simulink model "sim_sil_target_TrapezoidalCommutation_s32k1xx"  (Simulink 9.0)
settings: Solver=FixedStepDiscrete  StartTime=0.0  StopTime=12  FixedStep=1  RelTol=1e-3  EnableMultiTasking=on
InitFcn:
  | mbd_s32k_consistency_checks(bdroot(gcs));
undefined symbols (not defined in the file): LQFP
libraries: mbd_s32k1xx_ec_toolbox x1
settings Model: Creator=NXP MBDT Team  LastModifiedBy=nxf35172
settings DataIOCC: ExternalInput=off  InitialState=off  LimitDataPoints=on  SaveOutput=off  SignalLogging=off  SaveTime=off
settings OptimizationCC: DefaultParameterBehavior=Inlined  EnhancedBackFolding=on  PassReuseOutputArgsAs=Individual arguments  LifeSpan=auto  OptimizeBlockOrder=speed  DifferentSizesBufferReuse=on
settings DebuggingCC: UnderspecifiedInitializationDetection=Simplified  MergeDetectMultiDrivingBlocksExec=error  SolverPrmCheckMsg=warning  InheritedTsInSrcMsg=none  SingleTaskRateTransMsg=error  ParameterTunabilityLossMsg=error  UnconnectedInputMsg=error  UnconnectedOutputMsg=error  UnconnectedLineMsg=error  AllowSymbolicDim=off  UnknownTsInhSupMsg=error
settings HardwareCC: ProdIntDivRoundTo=Zero  ProdEndianess=LittleEndian  ProdHWDeviceType=Generic->Custom
settings SFSimCC: MATLABDynamicMemAlloc=off
settings RTWCC: SystemTargetFile=mbd_s32k.tlc  MakeCommand=mbd_s32k_make_rtw COPY_MDLREF_INCLUDES=0  TemplateMakefile=mbd_s32k.tmf  Description=Model Based Design Toolbox S32K1xx Code Generation Target  GenerateReport=on  IncludeHyperlinkInReport=on  LaunchReport=on  PortableWordSizes=on  GenerateTraceInfo=on  GenerateTraceReport=on  GenerateTraceReportSl=on  GenerateTraceReportSf=on  GenerateTraceReportEml=on
settings CodeAppCC: ForceParamTrailComments=on  IgnoreCustomStorageClasses=off  MaxIdLength=63  OperatorAnnotations=on  SimulinkDataObjDesc=on  SFDataObjDesc=on  InsertBlockDesc=on  StateflowObjectComments=off
settings STFCustomTargetCC: MultiwordLength=256  GenerateSampleERTMain=on  CombineOutputUpdateFcns=on  SuppressErrorStatus=on  ERTCustomFileBanners=on  SupportAbsoluteTime=off  SupportContinuousTime=off  SupportNonInlinedSFcns=off  RemoveResetFunc=on  MATLABClassNameForMDSCustomization=Simulink.SoftwareTarget.ERTCustomization  GRTInterface=off  SystemTargetFile=mbd_s32k.tlc
settings ERTTargetCC: GenerateSampleERTMain=on  ParMdlRefBuildCompliant=off  CompOptLevelCompliant=off  ConcurrentExecutionCompliant=off  SuppressErrorStatus=on  SupportAbsoluteTime=off  ModelStepFunctionPrototypeControlCompliant=off  CPPClassGenCompliant=off  UseToolchainInfoCompliant=off  InlinedParameterPlacement=NonHierarchical  ERTCustomFileTemplate=example_file_process.tlc

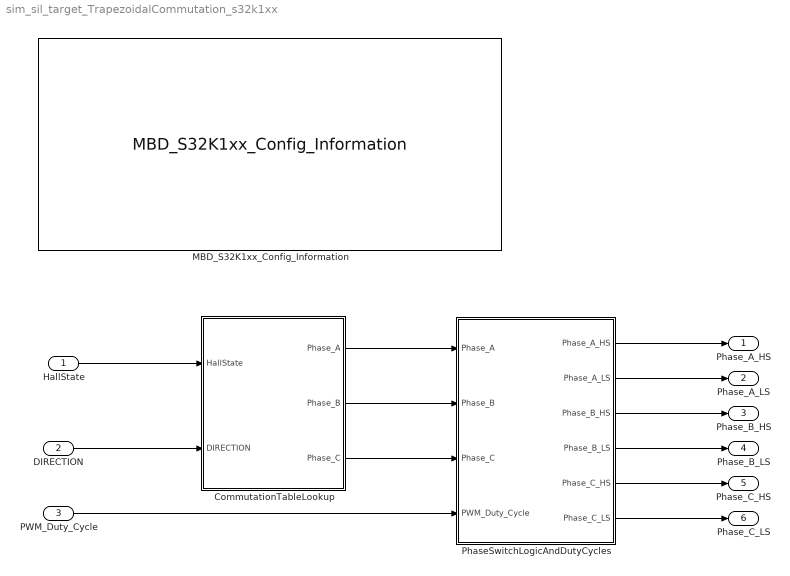
== system sim_sil_target_TrapezoidalCommutation_s32k1xx ==
  HallState : Inport
  DIRECTION : Inport  Port=2
  PWM_Duty_Cycle : Inport  Port=3
  CommutationTableLookup : Stateflow chart  TreatAsAtomicUnit=on
  MBD_S32K1xx_Config_Information : mbd_s32k1xx_ec_toolbox/MBD_S32K1xx_Config_Information  mbdt_ver=0  disp_str=|  config_params=target_mcu::S32K144-64KB_SRAM;;mcu_target_package::100-pin;;mcu_system_clock_freq::80;;mcu_xtal_freq::External 8;;mcu_steptick_timer::LPIT Channel 0;;mcu_steptick_prio::15;;ds_import_enable::on;;target_compiler::GCC;;target_memory::FLASH;;gcc_target_compile_opts::-c -mcpu=cortex-m4 -mthumb -mfloat-abi=hard -mfpu=fpv4-sp-d16 -O1 -g -gstrict-dwarf;;gcc_target_assemble_opts::-mcpu=cortex-m4 -mthumb -mfloat-abi=hard -mfpu=fpv4-sp-d16 -g;;gcc_target_link_opts::-mcpu=cortex-m4 -mthumb -mfloat-abi=hard -mfpu=fpv4-sp-d16;;gcc_target_lib_opts::;;gcc_target_default_lcf::on;;gcc_target_user_lcf::S32K144_64_flash.ld;;ghs_target_compile_opts::-cpu=cortexm4f -thumb -fpu=vfpv4_d16 -fsingle -Ogeneral -Wundef -Wimplicit-int -Wshadow -Wtrigraphs --no_commons --gnu_asm -gnu99 -gdwarf-2 -G ;;ghs_target_assemble_opts::-cpu=cortexm4f -fpu=vfpv4_d16;;ghs_target_link_opts::-cpu=cortexm4f -thumb -fpu=vfpv4_d16;;ghs_target_lib_opts::;;ghs_target_default_lcf::on;;ghs_target_user_lcf::S32K144_64_flash.ld;;iar_target_compile_opts::--cpu=Cortex-M4F --thumb --fpu=VFPv4_sp -Ol -e --debug --dlib_config normal;;iar_target_assemble_opts::--cpu Cortex-M4F --thumb --fpu VFPv4_sp;;iar_target_link_opts::--no_exceptions --vfe --inline;;iar_target_lib_opts::;;iar_target_default_lcf::on;;iar_target_user_lcf::S32K144_64_flash.icf;;pil_download_enable::on;;rbl_download_enable::off;;rbl_restart_request::off;;rbl_start_delay::5000000;;rbl_com_port::1;;pil_download_rate::57600;;rbl_download_interface::OpenSDA;;pil_opensda_drive::E;;ModelRef_PcrCheckEnDis::on;;ADC_PcrCheckEnDis::on;;AMMCLIB_PcrCheckEnDis::on;;CMP_PcrCheckEnDis::on;;CSEc_PcrCheckEnDis::on;;FlexCAN_PcrCheckEnDis::on;;FlexIO_PcrCheckEnDis::on;;FM_PcrCheckEnDis::on;;FTM_Independent_Ouputs_PcrCheckEnDis::on;;FTM_Complementary_Ouputs_PcrCheckEnDis::on;;FTM_Three_Phase_Outputs_PcrCheckEnDis::on;;FTM_Input_Edge_Inputs_PcrCheckEnDis::on;;FTM_Dual_Edge_Inputs_PcrCheckEnDis::on;;FTM_Quadrature_Inputs_PcrCheckEnDis::on;;GPIO_OutputPcrCheckEnDis::on;;GPIO_InputPcrCheckEnDis::on;;LPI2C_PcrCheckEnDis::on;;LPSPI_PcrCheckEnDis::on;;LPTMR_PcrCheckEnDis::on;;LPUART_PcrCheckEnDis::on;;PDB0_PcrCheckEnDis::on;;PIT_PcrCheckEnDis::on;;Profile_PcrCheckEnDis::on;;  mcu_target_name=S32K144  mcu_target_package=100-LQFP  mcu_target_sram_size=48KB  mcu_system_clock_freq=80  mcu_xtal_freq=External 8  mcu_steptick_timer=LPIT Channel 0  mcu_steptick_prio=15  ds_import_enable=on  target_compiler=GCC  target_memory=FLASH  gcc_target_compile_opts=-mcpu=cortex-m4 -mthumb -mfloat-abi=hard -mfpu=fpv4-sp-d16 -O1 -g -gstrict-dwarf  gcc_target_assemble_opts=-mcpu=cortex-m4 -mthumb -mfloat-abi=hard -mfpu=fpv4-sp-d16 -g  gcc_target_link_opts=-mcpu=cortex-m4 -mthumb -mfloat-abi=hard -mfpu=fpv4-sp-d16  gcc_target_default_lcf=on  gcc_target_user_lcf=S32K144_48_flash.ld  ghs_target_compile_opts=-cpu=cortexm4f -thumb -DARM_MATH_CM4 -fpu=vfpv4_d16 -fsingle -Ogeneral -Wundef -Wimplicit-int -Wshadow -Wtrigraphs --no_commons --gnu_asm -gnu99 -gdwarf-2 -G  ghs_target_assemble_opts=-cpu=cortexm4f -fpu=vfpv4_d16  ghs_target_link_opts=-cpu=cortexm4f -thumb -fpu=vfpv4_d16  ghs_target_default_lcf=off  ghs_target_user_lcf=S32K144_48_flash.ld  iar_target_compile_opts=--cpu=Cortex-M4F --thumb --fpu=VFPv4_sp -Ol -e --debug --dlib_config normal  iar_target_assemble_opts=--cpu Cortex-M4F --thumb --fpu VFPv4_sp  iar_target_link_opts=--no_exceptions --vfe --inline  iar_target_default_lcf=off  iar_target_user_lcf=S32K144_48_flash.icf  pil_download_enable=off  rbl_download_enable=off  rbl_start_delay=5000000  rbl_download_interface=OpenSDA  rbl_restart_request=off  rbl_com_port=Custom  rbl_com_port_custom=COM1  pil_download_rate=57600  pil_opensda_drive=Custom  pil_opensda_drive_custom=D  pil_uart_instance=0  pil_uart_rx=PTA2: [LPUART0_RX | Receive]  pil_uart_tx=PTA3: [LPUART0_TX | Transmit]  FTM_PWM_PcrCheckEnDis=on  FTM_Input_Edge_Inputs_PcrCheckEnDis=on  FTM_Dual_Edge_Inputs_PcrCheckEnDis=on  FTM_Quadrature_Inputs_PcrCheckEnDis=on  FTM_Hall_Sensor_Inputs_PcrCheckEnDis=on  LPTMR_PcrCheckEnDis=on  PIT_PcrCheckEnDis=on  RTC_PcrCheckEnDis=on  FlexCAN_PcrCheckEnDis=on  LIN_PcrCheckEnDis=on  FlexIO_PcrCheckEnDis=on  LPI2C_PcrCheckEnDis=on  LPSPI_PcrCheckEnDis=on  LPUART_PcrCheckEnDis=on  CMP_PcrCheckEnDis=on  GPIO_OutputPcrCheckEnDis=on  GPIO_InputPcrCheckEnDis=on  SBC_PcrCheckEnDis=on  AMMCLIB_PcrCheckEnDis=on  FM_PcrCheckEnDis=on  Profile_PcrCheckEnDis=on  ConfigParams_PcrCheckEnDis=on  ModelRef_PcrCheckEnDis=on  PDB0_PcrCheckEnDis=on  CSEc_PcrCheckEnDis=on  eDMA_PcrCheckEnDis=on  ADC_PcrCheckEnDis=on  WDOG_PcrCheckEnDis=on
      | Target : S32K144-64KB_SRAM
      | Package : 100-pin
      | System clock : 80 MHz
      | XTAL clock : External 8 MHz
      | Compiler : GCC
      | Target Type : FLASH
      | Processor-In-Loop : (COM1, 57600, OpenSDA: E)
      | Step Tick Interrupt Priority : 15
  PhaseSwitchLogicAndDutyCycles : Stateflow chart  TreatAsAtomicUnit=on
  Phase_A_HS : Outport
  Phase_A_LS : Outport  Port=2
  Phase_B_HS : Outport  Port=3
  Phase_B_LS : Outport  Port=4
  Phase_C_HS : Outport  Port=5
  Phase_C_LS : Outport  Port=6
  wires:
  PhaseSwitchLogicAndDutyCycles/2(Phase_A_LS) -> Phase_A_LS/1
  PhaseSwitchLogicAndDutyCycles/1(Phase_A_HS) -> Phase_A_HS/1
  CommutationTableLookup/3(Phase_C) -> PhaseSwitchLogicAndDutyCycles/3(Phase_C)
  PhaseSwitchLogicAndDutyCycles/3(Phase_B_HS) -> Phase_B_HS/1
  PhaseSwitchLogicAndDutyCycles/4(Phase_B_LS) -> Phase_B_LS/1
  HallState/1 -> CommutationTableLookup/1(HallState)
  CommutationTableLookup/2(Phase_B) -> PhaseSwitchLogicAndDutyCycles/2(Phase_B)
  PWM_Duty_Cycle/1 -> PhaseSwitchLogicAndDutyCycles/4(PWM_Duty_Cycle)
  CommutationTableLookup/1(Phase_A) -> PhaseSwitchLogicAndDutyCycles/1(Phase_A)
  PhaseSwitchLogicAndDutyCycles/6(Phase_C_LS) -> Phase_C_LS/1
  PhaseSwitchLogicAndDutyCycles/5(Phase_C_HS) -> Phase_C_HS/1
  DIRECTION/1 -> CommutationTableLookup/2(DIRECTION)

== stateflow chart CommutationTableLookup ==
  (junction 11) -> (junction 10) [order 1] : /*If Direction is Negative */
      | [DIRECTION < 0]
  (default) -> (junction 11)
  (junction 10) -> (junction 12) : {
      |    Phase_A = ccwTable[HallState][0];
      |    Phase_B = ccwTable[HallState][1];
      |    Phase_C = ccwTable[HallState][2];
      | }
  (junction 11) -> (junction 13) [order 2] : {
      |    Phase_A = cwTable[HallState][0];
      |    Phase_B = cwTable[HallState][1];
      |    Phase_C = cwTable[HallState][2];
      | }
  (junction 13) -> (junction 12)
  data: cwTable constant uint8 size=[8 3] =[0 0 0; 2 1 0; 0 2 1; 2 0 1; 1 0 2; 0 1 2; 1 2 0; 0 0 0]; HallState input uint8; Phase_A output uint8; Phase_B output uint8; Phase_C output uint8; ccwTable constant uint8 size=[8 3] =[0 0 0; 1 2 0; 0 1 2; 1 0 2; 2 0 1; 0 2 1; 2 1 0; 0 0 0]; DIRECTION input single

== stateflow chart PhaseSwitchLogicAndDutyCycles ==
  settings: sampleTime=0.500
  note: Phase States:
      | 0 = NC
      | 1 = -Vdcb
      | 2 = +Vdcb
  (default) -> (junction 32)
  (junction 32) -> (junction 33) [order 1] : /*check for phase state 0 */
      | [Phase_A == 0]
      | /*set output for state 0 */
      | {Phase_A_HS = 0; Phase_A_LS =0;}
  (junction 32) -> (junction 34) [order 2]
  (junction 33) -> (junction 35)
  (junction 34) -> (junction 35) [order 1] : /*check for phase state 1 */
      | [Phase_A == 1]
      | /*set output for state 1 */
      | {Phase_A_HS = 0; Phase_A_LS = PWM_Duty_Cycle;}
  (junction 34) -> (junction 36) [order 2]
  (junction 35) -> (junction 37)
  (junction 36) -> (junction 37) [order 1] : /*check for phase state 2 */
      | [Phase_A == 2]
      | /*set output for state 2 */
      | {Phase_A_HS = 1; Phase_A_LS = 0;}
  (junction 36) -> (junction 38) [order 2]
  (junction 37) -> (junction 39)
  (junction 38) -> (junction 39)
  (junction 39) -> (junction 40) [order 1] : /*check for phase state 0 */
      | [Phase_B == 0]
      | /*set output for state 0 */
      | {Phase_B_HS = 0; Phase_B_LS = 0;}
  (junction 39) -> (junction 41) [order 2]
  (junction 40) -> (junction 42)
  (junction 41) -> (junction 42) [order 1] : /*check for phase state 1 */
      | [Phase_B == 1]
      | /*set output for state 1 */
      | {Phase_B_HS = 0; Phase_B_LS = PWM_Duty_Cycle;}
  (junction 41) -> (junction 43) [order 2]
  (junction 42) -> (junction 44)
  (junction 43) -> (junction 44) [order 1] : /*check for phase state 2 */
      | [Phase_B == 2]
      | /*set output for state 2 */
      | {Phase_B_HS = 1; Phase_B_LS = 0;}
  (junction 43) -> (junction 45) [order 2]
  (junction 44) -> (junction 46)
  (junction 45) -> (junction 46)
  (junction 46) -> (junction 47) [order 1] : /*check for phase state 0 */
      | [Phase_C == 0]
      | /*set output for state 0 */
      | {Phase_C_HS = 0; Phase_C_LS = 0;}
  (junction 46) -> (junction 48) [order 2]
  (junction 47) -> (junction 49)
  (junction 48) -> (junction 49) [order 1] : /*check for phase state 1 */
      | [Phase_C == 1]
      | /*set output for state 1 */
      | {Phase_C_HS = 0; Phase_C_LS = PWM_Duty_Cycle;}
  (junction 48) -> (junction 50) [order 2]
  (junction 49) -> (junction 51)
  (junction 50) -> (junction 51) [order 1] : /*check for phase state 2 */
      | [Phase_C == 2]
      | /*set output for state 2 */
      | {Phase_C_HS = 1; Phase_C_LS = 0;}
  (junction 50) -> (junction 52) [order 2]
  (junction 51) -> (junction 53)
  (junction 52) -> (junction 53)
  data: Phase_A input uint8; Phase_B input uint8; Phase_C input uint8; Phase_A_HS output single; Phase_A_LS output single; Phase_B_HS output single; Phase_B_LS output single; Phase_C_HS output single; Phase_C_LS output single; PWM_Duty_Cycle input single [0..100]
